simulink model "PIDplusPlant"  (R2014a)
settings: Solver=ode45  StartTime=0.0  StopTime=100  RelTol=1e-3
settings Model: Creator=HP  LastModifiedBy=HP

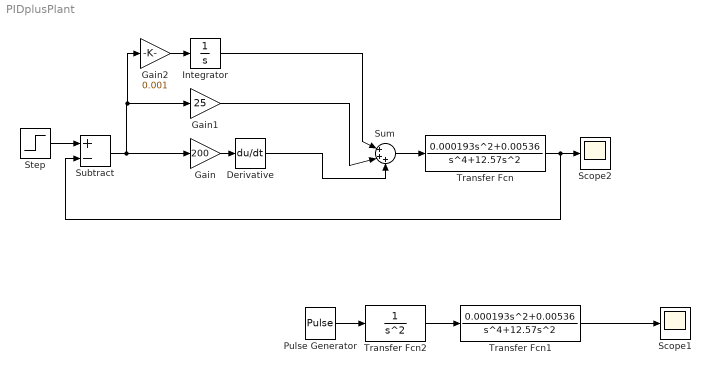
== system PIDplusPlant ==
  Derivative : Derivative
  Gain : Gain  Gain=200
  Gain1 : Gain  Gain=25
  Gain2 : Gain  Gain=0.001
  Integrator : Integrator
  Pulse Generator : DiscretePulseGenerator  PulseType=Time based  Amplitude=30  Period=1/1000  PulseWidth=85
  Scope1 : Scope
      settings: MaxDataPoints=20000
  Scope2 : Scope
      settings: TimeRange=100  YMin=0.9400000000000001  YMax=1.08  MaxDataPoints=20000
  Step : Step  SampleTime=0
  Subtract : Sum  Inputs=+-
  Sum : Sum  Inputs=|+++
  Transfer Fcn : TransferFcn  Numerator=[0.000193 0 0.00536]  Denominator=[1 0 12.57 0 0]
  Transfer Fcn1 : TransferFcn  Numerator=[0.000193 0 0.00536]  Denominator=[1 0 12.57 0 0]
  Transfer Fcn2 : TransferFcn  Denominator=[1 0 0]
  wires:
  Transfer Fcn/1 -> Subtract/2, Scope2/1
  Step/1 -> Subtract/1
  Subtract/1 -> Gain2/1, Gain1/1, Gain/1
  Gain/1 -> Derivative/1
  Derivative/1 -> Sum/3
  Gain1/1 -> Sum/2
  Integrator/1 -> Sum/1
  Sum/1 -> Transfer Fcn/1
  Gain2/1 -> Integrator/1
  Pulse Generator/1 -> Transfer Fcn2/1
  Transfer Fcn1/1 -> Scope1/1
  Transfer Fcn2/1 -> Transfer Fcn1/1
